simulink model "robotarm"  (R2024a)
settings: Solver=VariableStepAuto  StartTime=0.0  StopTime=10.0  RelTol=1e-3
settings Model: Creator=max11mus  LastModifiedBy=max11mus
settings DataIOCC: ReturnWorkspaceOutputs=off

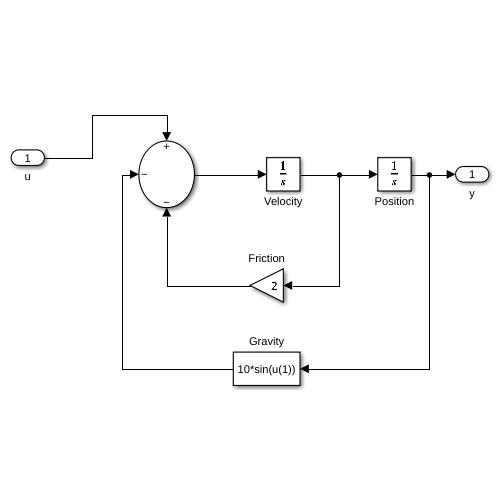
[thumbnail: Simulink's stored preview of the top-level diagram]
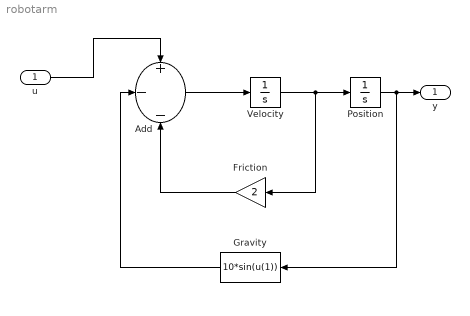
== system robotarm ==
  u : Inport
  Add : Sum  Inputs=+||-||-
  Friction : Gain  Gain=2
  Gravity : Fcn  Expr=10*sin(u(1))
  Position : Integrator
  Velocity : Integrator
  y : Outport
  wires:
  u/1 -> Add/1
  Add/1 -> Velocity/1
  Velocity/1 -> Friction/1, Position/1
  Position/1 -> Gravity/1, y/1
  Friction/1 -> Add/3
  Gravity/1 -> Add/2
